simulink model "SbW_can_Add"  (R2023b)
settings: Solver=VariableStepAuto  StartTime=0.0  StopTime=60  RelTol=1e-3
model workspace (MAT data in the model file):
  x = 4
undefined symbols (not defined in the file): canChannel
libraries: canlib x13, canmsglib x10, simulink x5
settings Model: Creator=jcm52  LastModifiedBy=jcm52
settings DebuggingCC: ParameterPrecisionLossMsg=none

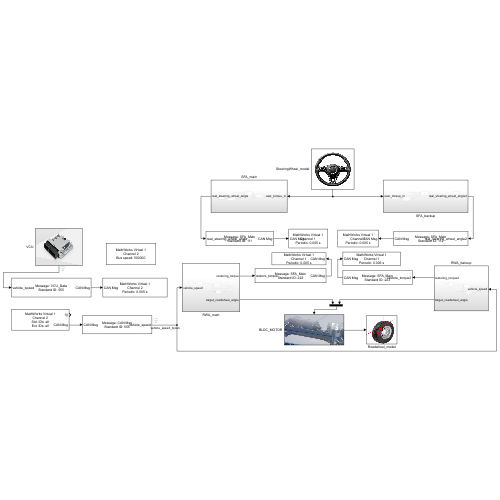
[thumbnail: Simulink's stored preview of the top-level diagram]
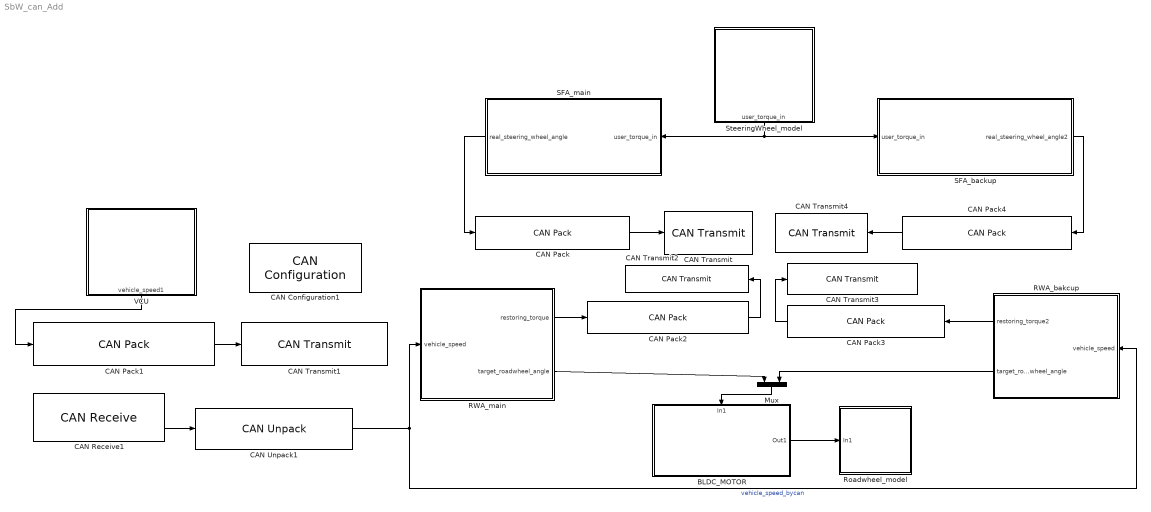
== system SbW_can_Add ==
  BLDC_MOTOR : Subsystem
      settings: PortSchema="{\"entries\":[{\"content\":{\"sides\":[{\"content\":{\"connectorIds\":[\"In1\"]},\"type\":\"ConnectorPlacement.EquallySpacedRectSide\",\"uuid\":\"0edd4ca9-6ba3-44cf-84e8-411fcbfa08a9\"},{\"content\":{\"side\":\"RIGHT\"},\"type\":\"ConnectorPlacement.EquallySpacedRectSide\",\"uuid\":\"1b1e5137-5b53-47d6-9c75-eac4291ecae6\"},{\"content\":{\"side\":\"TOP\"},\"type\":\"ConnectorPlacement.EquallySpacedRectSide\",\"uuid\":\"e92c0db8-e45c-4a10-9453-9421a3afd429\"},{\"content\":{\"connectorIds\":[\"Out1\"],\"side\":\"BOTTOM\"},\"type\":\"ConnectorPlacement.EquallySpacedRectSide\",\"uuid\":\"36596678-497e-4525-9553-fa484b150962\"}]},\"type\":\"ConnectorPlacement.EquallySpacedConnector\",\"uuid\":\"01756abd-94b0-4550-bc67-6fd2a819bbbe\"}],\"packageUris\":[\"http://schema.mathworks.com/mf0/Connector/R2020b\"],\"version\":\"1.0\"}"
      mask Display: image('image\bldc_motor.jpg');
  CAN Configuration1 : canlib/CAN Configuration  BlockHandle=2.0007  Device=MathWorks Virtual 1 (Channel 2)  DeviceMenu=MathWorks Virtual 1 (Channel 2)  ObjConstructor=canChannel('MathWorks', 'Virtual 1', 2)  BusSpeed=500000  EnableBitParameters=off  AckMode=Normal
  CAN Pack : canmsglib/CAN Pack  MsgList=(none)  MsgName=SFA_Main  MsgIDType=Standard (11-bit identifier)  MsgIdentifier=111  MsgLength=8  Remote=off  ApplyMinMax=off  BusOutput=off  SignalInfo={ 'real_steering_wheel_angle', '0', '32', 'LE', 'single', 'Standard', '0', '1', '0', '-4', '4' }
      settings: LibrarySourceBlock=canlib/CAN Pack  DataFormat=manually specified signals
  CAN Pack1 : canmsglib/CAN Pack  MsgList=(none)  MsgName=VCU_Data  MsgIDType=Standard (11-bit identifier)  MsgIdentifier=555  MsgLength=8  Remote=off  ApplyMinMax=off  BusOutput=off  SignalInfo={ 'vehicle_speed', '0', '16', 'LE', 'unsigned', 'Standard', '0', '1', '0', '-Inf', 'Inf' }
      settings: LibrarySourceBlock=canlib/CAN Pack  DataFormat=manually specified signals
  CAN Pack2 : canmsglib/CAN Pack  MsgList=(none)  MsgName=SFA_Main  MsgIDType=Standard (11-bit identifier)  MsgIdentifier=222  MsgLength=8  Remote=off  ApplyMinMax=off  BusOutput=off  SignalInfo={ 'restore_torque', '0', '32', 'LE', 'single', 'Standard', '0', '1', '0', '-10', '10' }
      settings: LibrarySourceBlock=canlib/CAN Pack  DataFormat=manually specified signals
  CAN Pack3 : canmsglib/CAN Pack  MsgList=(none)  MsgName=SFA_Main  MsgIDType=Standard (11-bit identifier)  MsgIdentifier=223  MsgLength=8  Remote=off  ApplyMinMax=off  BusOutput=off  SignalInfo={ 'restore_torque2', '0', '32', 'LE', 'single', 'Standard', '0', '1', '0', '-10', '10' }
      settings: LibrarySourceBlock=canlib/CAN Pack  DataFormat=manually specified signals
  CAN Pack4 : canmsglib/CAN Pack  MsgList=(none)  MsgName=SFA_Main  MsgIDType=Standard (11-bit identifier)  MsgIdentifier=112  MsgLength=8  Remote=off  ApplyMinMax=off  BusOutput=off  SignalInfo={ 'real_steering_wheel_angle2', '0', '32', 'LE', 'single', 'Standard', '0', '1', '0', '-4', '4' }
      settings: LibrarySourceBlock=canlib/CAN Pack  DataFormat=manually specified signals
  CAN Receive1 : canlib/CAN Receive  BlockHandle=9.0007  Device=MathWorks Virtual 1 (Channel 2)  DeviceMenu=MathWorks Virtual 1 (Channel 2)  ObjConstructor=canChannel('MathWorks', 'Virtual 1', 2)  EnableStandardIDsFilter=off  StdIDsCombo=Allow all  StandardIDs=0  EnableExtendedIDsFilter=off  ExtIDsCombo=Allow all  ExtendedIDs=0  SampleTime=0.005  MsgsPerTimestep=all  InternalFilterUpdateStatus=on  BusOutput=off
  CAN Transmit : canlib/CAN Transmit  BlockHandle=10.0007  Device=MathWorks Virtual 1 (Channel 1)  DeviceMenu=MathWorks Virtual 1 (Channel 1)  ObjConstructor=canChannel('MathWorks', 'Virtual 1', 1)  EnableEventTransmit=off  EnablePeriodicTransmit=on  MessagePeriod=0.005
  CAN Transmit1 : canlib/CAN Transmit  BlockHandle=11.0023  Device=MathWorks Virtual 1 (Channel 2)  DeviceMenu=MathWorks Virtual 1 (Channel 2)  ObjConstructor=canChannel('MathWorks', 'Virtual 1', 2)  EnableEventTransmit=off  EnablePeriodicTransmit=on  MessagePeriod=0.005
  CAN Transmit2 : canlib/CAN Transmit  BlockHandle=12.0007  Device=MathWorks Virtual 1 (Channel 1)  DeviceMenu=MathWorks Virtual 1 (Channel 1)  ObjConstructor=canChannel('MathWorks', 'Virtual 1', 1)  EnableEventTransmit=off  EnablePeriodicTransmit=on  MessagePeriod=0.005
  CAN Transmit3 : canlib/CAN Transmit  BlockHandle=13.0007  Device=MathWorks Virtual 1 (Channel 1)  DeviceMenu=MathWorks Virtual 1 (Channel 1)  ObjConstructor=canChannel('MathWorks', 'Virtual 1', 1)  EnableEventTransmit=off  EnablePeriodicTransmit=on  MessagePeriod=0.005
  CAN Transmit4 : canlib/CAN Transmit  BlockHandle=14.0009  Device=MathWorks Virtual 1 (Channel 1)  DeviceMenu=MathWorks Virtual 1 (Channel 1)  ObjConstructor=canChannel('MathWorks', 'Virtual 1', 1)  EnableEventTransmit=off  EnablePeriodicTransmit=on  MessagePeriod=0.005
  CAN Unpack1 : canmsglib/CAN Unpack  MsgList=(none)  MsgName=CAN Msg  MsgIDType=Standard (11-bit identifier)  MsgIdentifier=555  MsgLength=8  SignalInfo={ 'vehicle_speed', '0', '16', 'LE', 'unsigned', 'Standard', '0', '1', '0', '-Inf', 'Inf' }  IDPort=off  TimestampPort=off  ErrorPort=off  RemotePort=off  LengthPort=off  StatusPort=off  ApplyMinMax=off
      settings: LibrarySourceBlock=canlib/CAN Unpack
  Mux : Mux  Inputs=2
  RWA_bakcup : Subsystem
  RWA_main : Subsystem
  Roadwheel_model : Subsystem
      mask Display: image('image\road_wheel_angle.JPG');
  SFA_backup : Subsystem
  SFA_main : Subsystem
  SteeringWheel_model : Subsystem
      mask Display: image('image\pngtree-car-steering-wheel-png-image_13061877.png');
  VCU : Subsystem
      mask Display: image('image\vehicle-control-unit-compare-view-01_teaser.jpg');
  wires:
  SteeringWheel_model/1(user_torque_in) -> SFA_main/1(user_torque_in), SFA_backup/1(user_torque_in)
  CAN Pack1/1 -> CAN Transmit1/1
  CAN Receive1/2 -> CAN Unpack1/1
  CAN Unpack1/1 -> RWA_main/1(vehicle_speed), RWA_bakcup/1(vehicle_speed)  "vehicle_speed_bycan"
  VCU/1(vehicle_speed1) -> CAN Pack1/1
  SFA_main/1(real_steering_wheel_angle) -> CAN Pack/1
  CAN Pack/1 -> CAN Transmit/1
  CAN Pack4/1 -> CAN Transmit4/1
  SFA_backup/1(real_steering_wheel_angle2) -> CAN Pack4/1
  CAN Pack2/1 -> CAN Transmit2/1
  CAN Pack3/1 -> CAN Transmit3/1
  RWA_main/1(restoring_torque) -> CAN Pack2/1
  RWA_bakcup/1(restoring_torque2) -> CAN Pack3/1
  RWA_main/2(target_roadwheel_angle) -> Mux/1
  Mux/1 -> BLDC_MOTOR/1(In1)
  RWA_bakcup/2(target_roadwheel_angle) -> Mux/2
  BLDC_MOTOR/1(Out1) -> Roadwheel_model/1(In1)

== system SbW_can_Add/BLDC_MOTOR ==
  In1 : Inport
  Out1 : Outport

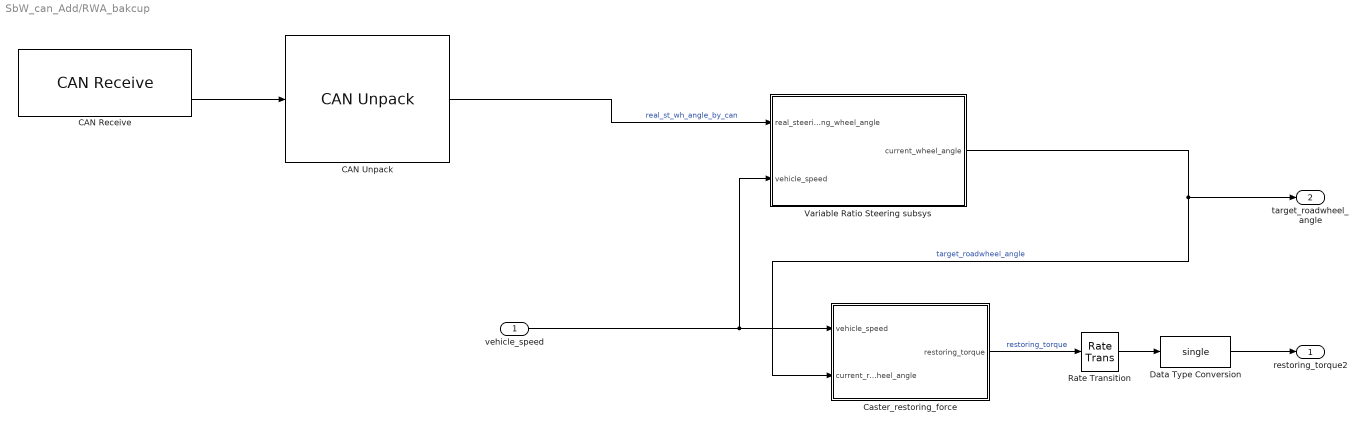
== system SbW_can_Add/RWA_bakcup ==
  vehicle_speed : Inport
  CAN Receive : canlib/CAN Receive  BlockHandle=20.0007  Device=MathWorks Virtual 1 (Channel 1)  DeviceMenu=MathWorks Virtual 1 (Channel 1)  ObjConstructor=canChannel('MathWorks', 'Virtual 1', 1)  EnableStandardIDsFilter=off  StdIDsCombo=Allow all  StandardIDs=0  EnableExtendedIDsFilter=off  ExtIDsCombo=Allow all  ExtendedIDs=0  SampleTime=0.005  MsgsPerTimestep=all  InternalFilterUpdateStatus=on  BusOutput=off
  CAN Unpack : canmsglib/CAN Unpack  MsgList=(none)  MsgName=CAN Msg  MsgIDType=Standard (11-bit identifier)  MsgIdentifier=111  MsgLength=8  SignalInfo={ 'real_steering_wheel_angle', '0', '32', 'LE', 'single', 'Standard', '0', '1', '0', '-4', '4' }  IDPort=off  TimestampPort=off  ErrorPort=off  RemotePort=off  LengthPort=off  StatusPort=off  ApplyMinMax=off
      settings: LibrarySourceBlock=canlib/CAN Unpack
  Caster_restoring_force : Subsystem
  Data Type Conversion : DataTypeConversion  OutDataTypeStr=single  SaturateOnIntegerOverflow=off  RndMeth=Floor
  Rate Transition : RateTransition  OutPortSampleTime=0.0001
  Variable Ratio Steering subsys : Subsystem
  restoring_torque2 : Outport
  target_roadwheel_angle : Outport  Port=2
  wires:
  Variable Ratio Steering subsys/1(current_wheel_angle) -> target_roadwheel_angle/1, Caster_restoring_force/2(current_roadwheel_angle)  "target_roadwheel_angle"
  vehicle_speed/1 -> Variable Ratio Steering subsys/2(vehicle_speed), Caster_restoring_force/1(vehicle_speed)
  Caster_restoring_force/1(restoring_torque) -> Rate Transition/1  "restoring_torque"
  CAN Unpack/1 -> Variable Ratio Steering subsys/1(real_steering_wheel_angle)  "real_st_wh_angle_by_can"
  CAN Receive/2 -> CAN Unpack/1
  Rate Transition/1 -> Data Type Conversion/1
  Data Type Conversion/1 -> restoring_torque2/1

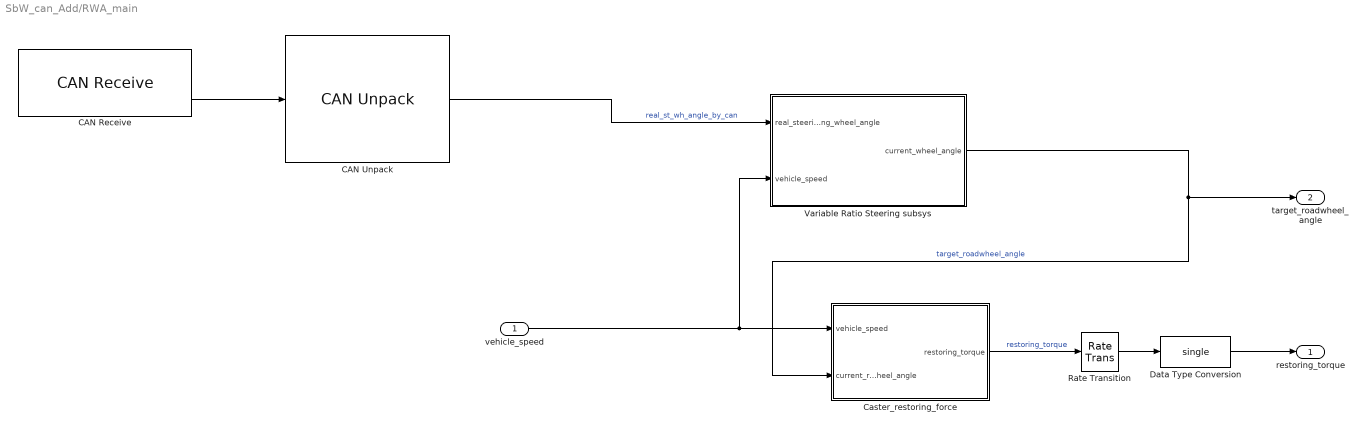
== system SbW_can_Add/RWA_main ==
  vehicle_speed : Inport
  CAN Receive : canlib/CAN Receive  BlockHandle=87.0007  Device=MathWorks Virtual 1 (Channel 1)  DeviceMenu=MathWorks Virtual 1 (Channel 1)  ObjConstructor=canChannel('MathWorks', 'Virtual 1', 1)  EnableStandardIDsFilter=off  StdIDsCombo=Allow all  StandardIDs=0  EnableExtendedIDsFilter=off  ExtIDsCombo=Allow all  ExtendedIDs=0  SampleTime=0.005  MsgsPerTimestep=all  InternalFilterUpdateStatus=on  BusOutput=off
  CAN Unpack : canmsglib/CAN Unpack  MsgList=(none)  MsgName=CAN Msg  MsgIDType=Standard (11-bit identifier)  MsgIdentifier=111  MsgLength=8  SignalInfo={ 'real_steering_wheel_angle', '0', '32', 'LE', 'single', 'Standard', '0', '1', '0', '-4', '4' }  IDPort=off  TimestampPort=off  ErrorPort=off  RemotePort=off  LengthPort=off  StatusPort=off  ApplyMinMax=off
      settings: LibrarySourceBlock=canlib/CAN Unpack
  Caster_restoring_force : Subsystem
  Data Type Conversion : DataTypeConversion  OutDataTypeStr=single  SaturateOnIntegerOverflow=off  RndMeth=Floor
  Rate Transition : RateTransition  OutPortSampleTime=0.0001
  Variable Ratio Steering subsys : Subsystem
  restoring_torque : Outport
  target_roadwheel_angle : Outport  Port=2
  wires:
  Variable Ratio Steering subsys/1(current_wheel_angle) -> target_roadwheel_angle/1, Caster_restoring_force/2(current_roadwheel_angle)  "target_roadwheel_angle"
  vehicle_speed/1 -> Variable Ratio Steering subsys/2(vehicle_speed), Caster_restoring_force/1(vehicle_speed)
  Caster_restoring_force/1(restoring_torque) -> Rate Transition/1  "restoring_torque"
  CAN Unpack/1 -> Variable Ratio Steering subsys/1(real_steering_wheel_angle)  "real_st_wh_angle_by_can"
  CAN Receive/2 -> CAN Unpack/1
  Rate Transition/1 -> Data Type Conversion/1
  Data Type Conversion/1 -> restoring_torque/1

== system SbW_can_Add/Roadwheel_model ==
  In1 : Inport

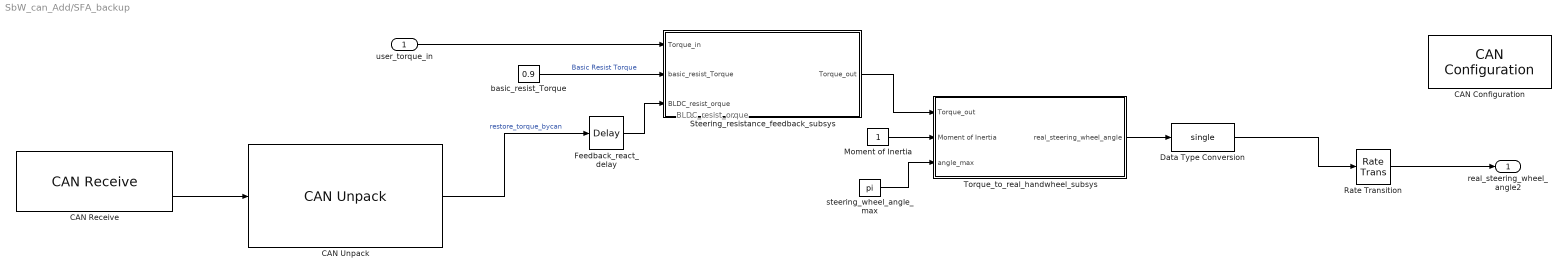
== system SbW_can_Add/SFA_backup ==
  note: BLDC_resist_orque
  user_torque_in : Inport
  CAN Configuration : canlib/CAN Configuration  BlockHandle=154.0007  Device=MathWorks Virtual 1 (Channel 1)  DeviceMenu=MathWorks Virtual 1 (Channel 1)  ObjConstructor=canChannel('MathWorks', 'Virtual 1', 1)  BusSpeed=250000  EnableBitParameters=off  AckMode=Normal
  CAN Receive : canlib/CAN Receive  BlockHandle=155.0013  Device=MathWorks Virtual 1 (Channel 1)  DeviceMenu=MathWorks Virtual 1 (Channel 1)  ObjConstructor=canChannel('MathWorks', 'Virtual 1', 1)  EnableStandardIDsFilter=off  StdIDsCombo=Allow all  StandardIDs=0  EnableExtendedIDsFilter=off  ExtIDsCombo=Allow all  ExtendedIDs=0  SampleTime=0.005  MsgsPerTimestep=all  InternalFilterUpdateStatus=on  BusOutput=off
  CAN Unpack : canmsglib/CAN Unpack  MsgList=(none)  MsgName=CAN Msg  MsgIDType=Standard (11-bit identifier)  MsgIdentifier=223  MsgLength=8  SignalInfo={ 'restore_torque', '0', '32', 'LE', 'single', 'Standard', '0', '1', '0', '-10', '10' }  IDPort=off  TimestampPort=off  ErrorPort=off  RemotePort=off  LengthPort=off  StatusPort=off  ApplyMinMax=off
      settings: LibrarySourceBlock=canlib/CAN Unpack
  Data Type Conversion : DataTypeConversion  OutDataTypeStr=single  SaturateOnIntegerOverflow=off  RndMeth=Floor
  Feedback_react_delay : TransportDelay  DelayTime=0.02
  Moment of Inertia : Constant
  Rate Transition : RateTransition  OutPortSampleTime=0.0001
  Steering_resistance_feedback_subsys : Subsystem
  Torque_to_real_handwheel_subsys : Subsystem
  basic_resist_Torque : Constant  Value=0.9  SampleTime=0.001
  steering_wheel_angle_max : Constant  Value=pi
  real_steering_wheel_angle2 : Outport
  wires:
  CAN Unpack/1 -> Feedback_react_delay/1  "restore_torque_bycan"
  Steering_resistance_feedback_subsys/1(Torque_out) -> Torque_to_real_handwheel_subsys/1(Torque_out)
  steering_wheel_angle_max/1 -> Torque_to_real_handwheel_subsys/3(angle_max)
  Torque_to_real_handwheel_subsys/1(real_steering_wheel_angle) -> Data Type Conversion/1
  Feedback_react_delay/1 -> Steering_resistance_feedback_subsys/3(BLDC_resist_orque)
  Moment of Inertia/1 -> Torque_to_real_handwheel_subsys/2(Moment of Inertia)
  user_torque_in/1 -> Steering_resistance_feedback_subsys/1(Torque_in)
  basic_resist_Torque/1 -> Steering_resistance_feedback_subsys/2(basic_resist_Torque)  "Basic Resist Torque"
  Data Type Conversion/1 -> Rate Transition/1
  Rate Transition/1 -> real_steering_wheel_angle2/1
  CAN Receive/2 -> CAN Unpack/1

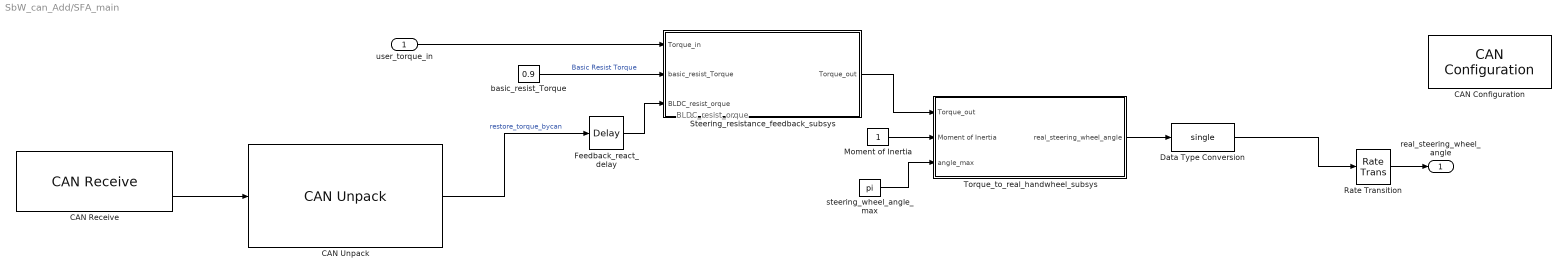
== system SbW_can_Add/SFA_main ==
  note: BLDC_resist_orque
  user_torque_in : Inport
  CAN Configuration : canlib/CAN Configuration  BlockHandle=272.0007  Device=MathWorks Virtual 1 (Channel 1)  DeviceMenu=MathWorks Virtual 1 (Channel 1)  ObjConstructor=canChannel('MathWorks', 'Virtual 1', 1)  BusSpeed=250000  EnableBitParameters=off  AckMode=Normal
  CAN Receive : canlib/CAN Receive  BlockHandle=273.0012  Device=MathWorks Virtual 1 (Channel 1)  DeviceMenu=MathWorks Virtual 1 (Channel 1)  ObjConstructor=canChannel('MathWorks', 'Virtual 1', 1)  EnableStandardIDsFilter=off  StdIDsCombo=Allow all  StandardIDs=0  EnableExtendedIDsFilter=off  ExtIDsCombo=Allow all  ExtendedIDs=0  SampleTime=0.005  MsgsPerTimestep=all  InternalFilterUpdateStatus=on  BusOutput=off
  CAN Unpack : canmsglib/CAN Unpack  MsgList=(none)  MsgName=CAN Msg  MsgIDType=Standard (11-bit identifier)  MsgIdentifier=222  MsgLength=8  SignalInfo={ 'restore_torque', '0', '32', 'LE', 'single', 'Standard', '0', '1', '0', '-10', '10' }  IDPort=off  TimestampPort=off  ErrorPort=off  RemotePort=off  LengthPort=off  StatusPort=off  ApplyMinMax=off
      settings: LibrarySourceBlock=canlib/CAN Unpack
  Data Type Conversion : DataTypeConversion  OutDataTypeStr=single  SaturateOnIntegerOverflow=off  RndMeth=Floor
  Feedback_react_delay : TransportDelay  DelayTime=0.02
  Moment of Inertia : Constant
  Rate Transition : RateTransition  OutPortSampleTime=0.0001
  Steering_resistance_feedback_subsys : Subsystem
  Torque_to_real_handwheel_subsys : Subsystem
  basic_resist_Torque : Constant  Value=0.9  SampleTime=0.001
  steering_wheel_angle_max : Constant  Value=pi
  real_steering_wheel_angle : Outport
  wires:
  CAN Unpack/1 -> Feedback_react_delay/1  "restore_torque_bycan"
  Steering_resistance_feedback_subsys/1(Torque_out) -> Torque_to_real_handwheel_subsys/1(Torque_out)
  steering_wheel_angle_max/1 -> Torque_to_real_handwheel_subsys/3(angle_max)
  Torque_to_real_handwheel_subsys/1(real_steering_wheel_angle) -> Data Type Conversion/1
  Feedback_react_delay/1 -> Steering_resistance_feedback_subsys/3(BLDC_resist_orque)
  Moment of Inertia/1 -> Torque_to_real_handwheel_subsys/2(Moment of Inertia)
  user_torque_in/1 -> Steering_resistance_feedback_subsys/1(Torque_in)
  basic_resist_Torque/1 -> Steering_resistance_feedback_subsys/2(basic_resist_Torque)  "Basic Resist Torque"
  Data Type Conversion/1 -> Rate Transition/1
  CAN Receive/2 -> CAN Unpack/1
  Rate Transition/1 -> real_steering_wheel_angle/1

== system SbW_can_Add/SteeringWheel_model ==
  Bias : Bias  Bias=-x  SaturateOnIntegerOverflow=off
  pulse_torque_in2 : DiscretePulseGenerator  PulseType=Time based  Amplitude=2*x  Period=5  PulseWidth=50
      mask Display: image('image\pngtree-car-steering-wheel-png-image_13061877.png');
  user_torque_in : Outport
  wires:
  pulse_torque_in2/1 -> Bias/1  "Torque_in"
  Bias/1 -> user_torque_in/1  "user_torque_in"

== system SbW_can_Add/VCU ==
  Data Type Conversion : DataTypeConversion  OutDataTypeStr=uint16  SaturateOnIntegerOverflow=off  RndMeth=Floor
  Rate Transition : RateTransition  OutPortSampleTime=0.001
  Subsystem : Subsystem
      mask Display: image('image\free-icon-speed-1455318.png');
  vehicle_speed1 : Outport
  wires:
  Subsystem/1(vehicle_speed1) -> Rate Transition/1
  Rate Transition/1 -> Data Type Conversion/1
  Data Type Conversion/1 -> vehicle_speed1/1

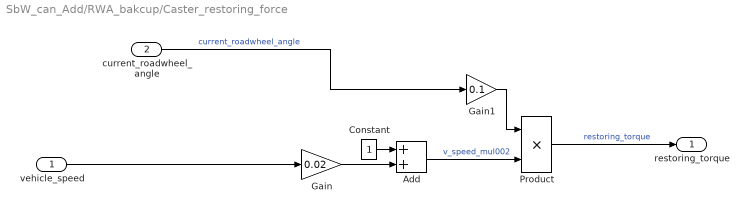
== system SbW_can_Add/RWA_bakcup/Caster_restoring_force ==
  vehicle_speed : Inport
  current_roadwheel_angle : Inport  Port=2
  Add : Sum
  Constant : Constant
  Gain : Gain  Gain=0.02
  Gain1 : Gain  Gain=0.1
  Product : Product
  restoring_torque : Outport
  wires:
  Gain/1 -> Add/2
  Constant/1 -> Add/1
  Add/1 -> Product/2  "v_speed_mul002"
  Gain1/1 -> Product/1
  Product/1 -> restoring_torque/1  "restoring_torque"
  current_roadwheel_angle/1 -> Gain1/1  "current_roadwheel_angle"
  vehicle_speed/1 -> Gain/1

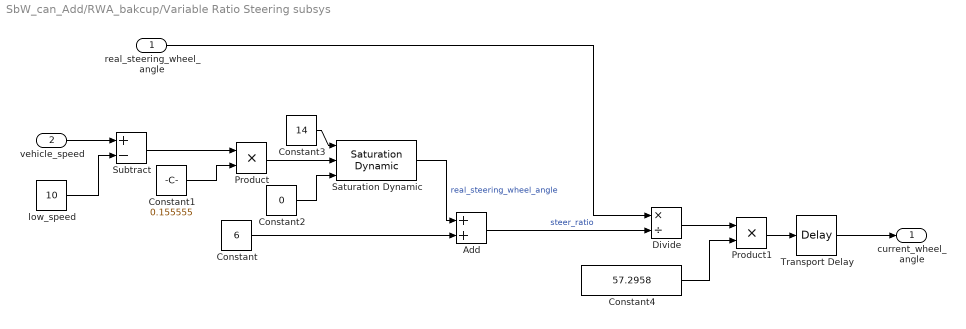
== system SbW_can_Add/RWA_bakcup/Variable Ratio Steering subsys ==
  real_steering_wheel_angle : Inport
  vehicle_speed : Inport  Port=2
  Add : Sum
  Constant : Constant  Value=6
  Constant1 : Constant  Value=0.155555
  Constant2 : Constant  Value=0
  Constant3 : Constant  Value=14
  Constant4 : Constant  Value=57.2958
  Divide : Product  Inputs=*/
  Product : Product
  Product1 : Product
  Saturation Dynamic : simulink/Discontinuities/Saturation Dynamic  OutMin=[]  OutMax=[]  OutDataTypeStr=double  OutDataType=fixdt(1, 16)  OutScaling=2^-10  DoSatur=off
  Subtract : Sum  Inputs=+-
  Transport Delay : TransportDelay  DelayTime=0.1
  low_speed : Constant  Value=10
  current_wheel_angle : Outport
  wires:
  vehicle_speed/1 -> Subtract/1
  low_speed/1 -> Subtract/2
  Subtract/1 -> Product/1
  Constant1/1 -> Product/2
  Constant/1 -> Add/2
  Product/1 -> Saturation Dynamic/2
  Constant2/1 -> Saturation Dynamic/3
  Constant3/1 -> Saturation Dynamic/1
  Saturation Dynamic/1 -> Add/1  "real_steering_wheel_angle"
  Add/1 -> Divide/2  "steer_ratio"
  real_steering_wheel_angle/1 -> Divide/1
  Divide/1 -> Product1/1
  Constant4/1 -> Product1/2
  Product1/1 -> Transport Delay/1
  Transport Delay/1 -> current_wheel_angle/1

== system SbW_can_Add/RWA_main/Caster_restoring_force ==
  vehicle_speed : Inport
  current_roadwheel_angle : Inport  Port=2
  Add : Sum
  Constant : Constant
  Gain : Gain  Gain=0.02
  Gain1 : Gain  Gain=0.1
  Product : Product
  restoring_torque : Outport
  wires:
  Gain/1 -> Add/2
  Constant/1 -> Add/1
  Add/1 -> Product/2  "v_speed_mul002"
  Gain1/1 -> Product/1
  Product/1 -> restoring_torque/1  "restoring_torque"
  current_roadwheel_angle/1 -> Gain1/1  "current_roadwheel_angle"
  vehicle_speed/1 -> Gain/1

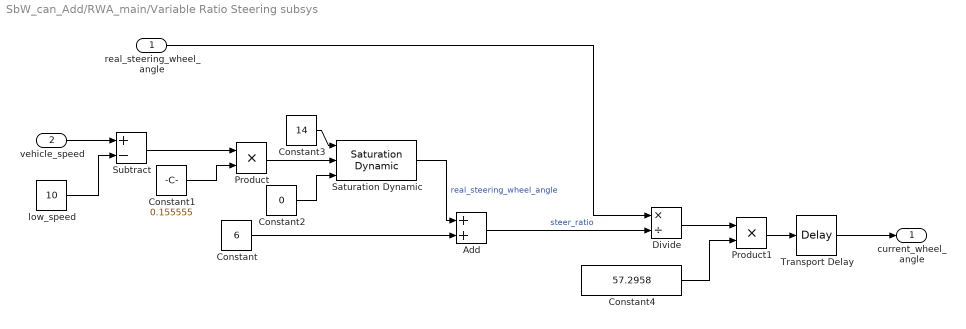
== system SbW_can_Add/RWA_main/Variable Ratio Steering subsys ==
  real_steering_wheel_angle : Inport
  vehicle_speed : Inport  Port=2
  Add : Sum
  Constant : Constant  Value=6
  Constant1 : Constant  Value=0.155555
  Constant2 : Constant  Value=0
  Constant3 : Constant  Value=14
  Constant4 : Constant  Value=57.2958
  Divide : Product  Inputs=*/
  Product : Product
  Product1 : Product
  Saturation Dynamic : simulink/Discontinuities/Saturation Dynamic  OutMin=[]  OutMax=[]  OutDataTypeStr=double  OutDataType=fixdt(1, 16)  OutScaling=2^-10  DoSatur=off
  Subtract : Sum  Inputs=+-
  Transport Delay : TransportDelay  DelayTime=0.1
  low_speed : Constant  Value=10
  current_wheel_angle : Outport
  wires:
  vehicle_speed/1 -> Subtract/1
  low_speed/1 -> Subtract/2
  Subtract/1 -> Product/1
  Constant1/1 -> Product/2
  Constant/1 -> Add/2
  Product/1 -> Saturation Dynamic/2
  Constant2/1 -> Saturation Dynamic/3
  Constant3/1 -> Saturation Dynamic/1
  Saturation Dynamic/1 -> Add/1  "real_steering_wheel_angle"
  Add/1 -> Divide/2  "steer_ratio"
  real_steering_wheel_angle/1 -> Divide/1
  Divide/1 -> Product1/1
  Constant4/1 -> Product1/2
  Product1/1 -> Transport Delay/1
  Transport Delay/1 -> current_wheel_angle/1

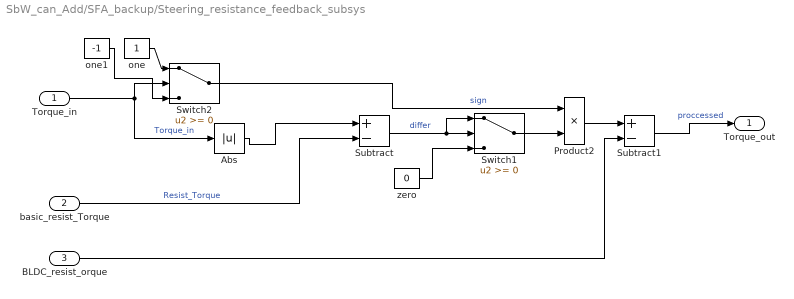
== system SbW_can_Add/SFA_backup/Steering_resistance_feedback_subsys ==
  Torque_in : Inport
  basic_resist_Torque : Inport  Port=2
  BLDC_resist_orque : Inport  Port=3
  Abs : Abs  SaturateOnIntegerOverflow=off
  Product2 : Product
  Subtract : Sum  Inputs=+-
  Subtract1 : Sum  Inputs=+-
  Switch1 : Switch  OutDataTypeStr=double  SaturateOnIntegerOverflow=off  InputSameDT=off
  Switch2 : Switch  OutDataTypeStr=double  SaturateOnIntegerOverflow=off  InputSameDT=off
  one : Constant
  one1 : Constant  Value=-1
  zero : Constant  Value=0
  Torque_out : Outport
  wires:
  Subtract/1 -> Switch1/1, Switch1/2  "differ"
  one/1 -> Switch2/1
  basic_resist_Torque/1 -> Subtract/2  "Resist_Torque"
  zero/1 -> Switch1/3
  Torque_in/1 -> Switch2/2, Abs/1  "Torque_in"
  Switch1/1 -> Product2/2
  Switch2/1 -> Product2/1  "sign"
  Abs/1 -> Subtract/1
  one1/1 -> Switch2/3
  BLDC_resist_orque/1 -> Subtract1/2
  Product2/1 -> Subtract1/1
  Subtract1/1 -> Torque_out/1  "proccessed"

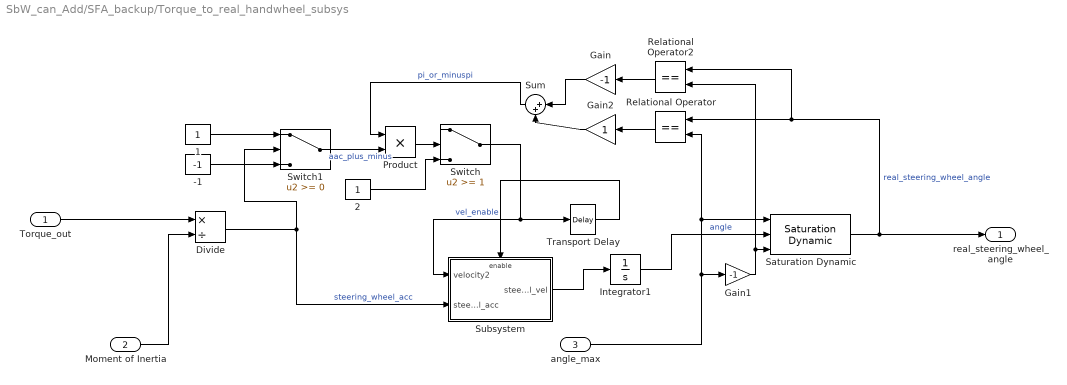
== system SbW_can_Add/SFA_backup/Torque_to_real_handwheel_subsys ==
  Torque_out : Inport
  Moment of Inertia : Inport  Port=2
  angle_max : Inport  Port=3
  -1 : Constant  Value=-1
  1 : Constant
  2 : Constant  OutDataTypeStr=boolean
  Divide : Product  Inputs=*/
  Gain : Gain  Gain=-1
  Gain1 : Gain  Gain=-1
  Gain2 : Gain
  Integrator1 : Integrator
  Product : Product
  Relational Operator : RelationalOperator  Operator===  OutDataTypeStr=boolean  RndMeth=Simplest  InputSameDT=off
  Relational Operator2 : RelationalOperator  Operator===  OutDataTypeStr=boolean  RndMeth=Simplest  InputSameDT=off
  Saturation Dynamic : simulink/Discontinuities/Saturation Dynamic  OutMin=[]  OutMax=[]  OutDataTypeStr=double  OutDataType=fixdt(1, 16)  OutScaling=2^-10  DoSatur=off
  Subsystem : Subsystem
  Sum : Sum  Inputs=|++
  Switch : Switch  Threshold=1  OutDataTypeStr=double  SaturateOnIntegerOverflow=off  InputSameDT=off
  Switch1 : Switch  SaturateOnIntegerOverflow=off  InputSameDT=off
  Transport Delay : TransportDelay  DelayTime=0.001
  real_steering_wheel_angle : Outport
  wires:
  Saturation Dynamic/1 -> Relational Operator2/1, Relational Operator/1, real_steering_wheel_angle/1  "real_steering_wheel_angle"
  Torque_out/1 -> Divide/1
  Integrator1/1 -> Saturation Dynamic/2  "angle"
  angle_max/1 -> Relational Operator/2, Saturation Dynamic/1, Gain1/1
  Gain1/1 -> Relational Operator2/2, Saturation Dynamic/3
  Moment of Inertia/1 -> Divide/2
  Divide/1 -> Switch1/2, Subsystem/2(steering_wheel_acc)  "steering_wheel_acc"
  Subsystem/1(steering_wheel_vel) -> Integrator1/1
  Switch/1 -> Subsystem/1(velocity2), Transport Delay/1  "vel_enable"
  Sum/1 -> Product/1  "pi_or_minuspi"
  -1/1 -> Switch1/3
  1/1 -> Switch1/1
  Switch1/1 -> Product/2  "aac_plus_minus"
  Relational Operator2/1 -> Gain/1
  Relational Operator/1 -> Gain2/1
  Gain/1 -> Sum/1
  Product/1 -> Switch/2
  2/1 -> Switch/3
  Gain2/1 -> Sum/2
  Transport Delay/1 -> Subsystem/Enable

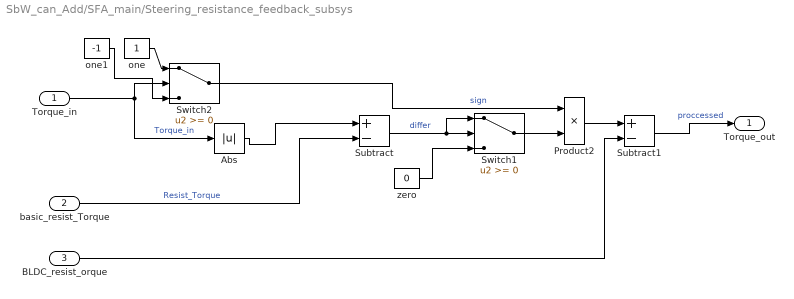
== system SbW_can_Add/SFA_main/Steering_resistance_feedback_subsys ==
  Torque_in : Inport
  basic_resist_Torque : Inport  Port=2
  BLDC_resist_orque : Inport  Port=3
  Abs : Abs  SaturateOnIntegerOverflow=off
  Product2 : Product
  Subtract : Sum  Inputs=+-
  Subtract1 : Sum  Inputs=+-
  Switch1 : Switch  OutDataTypeStr=double  SaturateOnIntegerOverflow=off  InputSameDT=off
  Switch2 : Switch  OutDataTypeStr=double  SaturateOnIntegerOverflow=off  InputSameDT=off
  one : Constant
  one1 : Constant  Value=-1
  zero : Constant  Value=0
  Torque_out : Outport
  wires:
  Subtract/1 -> Switch1/1, Switch1/2  "differ"
  one/1 -> Switch2/1
  basic_resist_Torque/1 -> Subtract/2  "Resist_Torque"
  zero/1 -> Switch1/3
  Torque_in/1 -> Switch2/2, Abs/1  "Torque_in"
  Switch1/1 -> Product2/2
  Switch2/1 -> Product2/1  "sign"
  Abs/1 -> Subtract/1
  one1/1 -> Switch2/3
  BLDC_resist_orque/1 -> Subtract1/2
  Product2/1 -> Subtract1/1
  Subtract1/1 -> Torque_out/1  "proccessed"

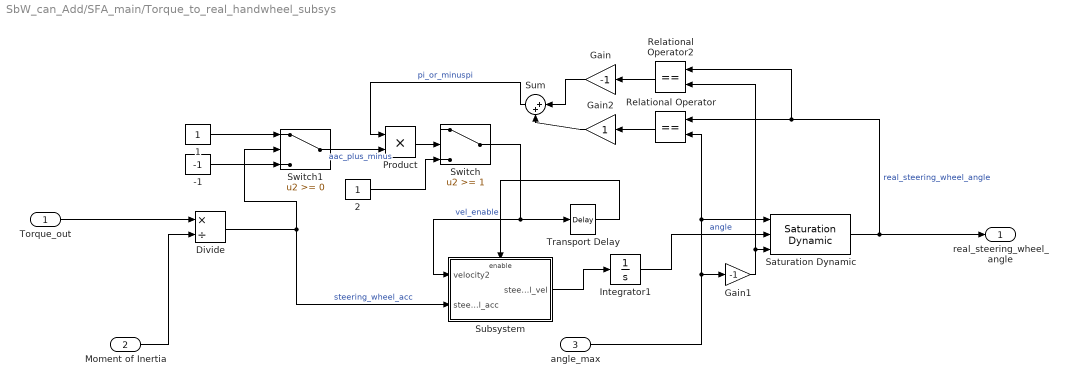
== system SbW_can_Add/SFA_main/Torque_to_real_handwheel_subsys ==
  Torque_out : Inport
  Moment of Inertia : Inport  Port=2
  angle_max : Inport  Port=3
  -1 : Constant  Value=-1
  1 : Constant
  2 : Constant  OutDataTypeStr=boolean
  Divide : Product  Inputs=*/
  Gain : Gain  Gain=-1
  Gain1 : Gain  Gain=-1
  Gain2 : Gain
  Integrator1 : Integrator
  Product : Product
  Relational Operator : RelationalOperator  Operator===  OutDataTypeStr=boolean  RndMeth=Simplest  InputSameDT=off
  Relational Operator2 : RelationalOperator  Operator===  OutDataTypeStr=boolean  RndMeth=Simplest  InputSameDT=off
  Saturation Dynamic : simulink/Discontinuities/Saturation Dynamic  OutMin=[]  OutMax=[]  OutDataTypeStr=double  OutDataType=fixdt(1, 16)  OutScaling=2^-10  DoSatur=off
  Subsystem : Subsystem
  Sum : Sum  Inputs=|++
  Switch : Switch  Threshold=1  OutDataTypeStr=double  SaturateOnIntegerOverflow=off  InputSameDT=off
  Switch1 : Switch  SaturateOnIntegerOverflow=off  InputSameDT=off
  Transport Delay : TransportDelay  DelayTime=0.001
  real_steering_wheel_angle : Outport
  wires:
  Saturation Dynamic/1 -> Relational Operator2/1, Relational Operator/1, real_steering_wheel_angle/1  "real_steering_wheel_angle"
  Torque_out/1 -> Divide/1
  Integrator1/1 -> Saturation Dynamic/2  "angle"
  angle_max/1 -> Relational Operator/2, Saturation Dynamic/1, Gain1/1
  Gain1/1 -> Relational Operator2/2, Saturation Dynamic/3
  Moment of Inertia/1 -> Divide/2
  Divide/1 -> Switch1/2, Subsystem/2(steering_wheel_acc)  "steering_wheel_acc"
  Subsystem/1(steering_wheel_vel) -> Integrator1/1
  Switch/1 -> Subsystem/1(velocity2), Transport Delay/1  "vel_enable"
  Sum/1 -> Product/1  "pi_or_minuspi"
  -1/1 -> Switch1/3
  1/1 -> Switch1/1
  Switch1/1 -> Product/2  "aac_plus_minus"
  Relational Operator2/1 -> Gain/1
  Relational Operator/1 -> Gain2/1
  Gain/1 -> Sum/1
  Product/1 -> Switch/2
  2/1 -> Switch/3
  Gain2/1 -> Sum/2
  Transport Delay/1 -> Subsystem/Enable

== system SbW_can_Add/VCU/Subsystem ==
  vehicle_speed : simulink/Sources/Repeating Sequence  rep_seq_t=[0 50 100]  rep_seq_y=[0 200 0]
  vehicle_speed1 : Outport
  wires:
  vehicle_speed/1 -> vehicle_speed1/1  "vehicle_speed"

== system SbW_can_Add/SFA_backup/Torque_to_real_handwheel_subsys/Subsystem ==
  velocity2 : Inport
  steering_wheel_acc : Inport  Port=2
  Enable : EnablePort  StatesWhenEnabling=reset
  Integrator : Integrator  ExternalReset=either
  steering_wheel_vel : Outport
  wires:
  Integrator/1 -> steering_wheel_vel/1  "steering_wheel_vel"
  velocity2/1 -> Integrator/2
  steering_wheel_acc/1 -> Integrator/1

== system SbW_can_Add/SFA_main/Torque_to_real_handwheel_subsys/Subsystem ==
  velocity2 : Inport
  steering_wheel_acc : Inport  Port=2
  Enable : EnablePort  StatesWhenEnabling=reset
  Integrator : Integrator  ExternalReset=either
  steering_wheel_vel : Outport
  wires:
  Integrator/1 -> steering_wheel_vel/1  "steering_wheel_vel"
  velocity2/1 -> Integrator/2
  steering_wheel_acc/1 -> Integrator/1
